simulink model "ForEach6"  (R2017b)
settings: Solver=ode3  StartTime=0.0  StopTime=10.0  FixedStep=0.200000  RelTol=1e-3  EnableMultiTasking=on
settings Model: Creator=hbourbou  LastModifiedBy=hbourbou
settings DataIOCC: LimitDataPoints=on  SaveFormat=Structure
settings OptimizationCC: LifeSpan=inf
settings DebuggingCC: SFUnexpectedBacktrackingDiag=warning  SFNoUnconditionalDefaultTransitionDiag=warning  SFExecutionAtInitializationDiag=none
settings HardwareCC: ProdBitPerPointer=32  ProdBitPerSizeT=32  ProdBitPerPtrDiffT=32  ProdLargestAtomicFloat=None  ProdIntDivRoundTo=Undefined  ProdEndianess=Unspecified  ProdWordSize=32  ProdHWDeviceType=32-bit Generic
settings ModelReferenceCC: PropagateSignalLabelsOutOfModel=off
settings CodeAppCC: StateflowObjectComments=on
settings GRTTargetCC: TargetLangStandard=C89/C90 (ANSI)  GeneratePreprocessorConditionals=Disable all
settings ConfigComp: CovMetricSettings=dw  CovHtmlReporting=on  CovSaveCumulativeToWorkspaceVar=on  CovSaveSingleToWorkspaceVar=on  CovExternalEMLEnable=off

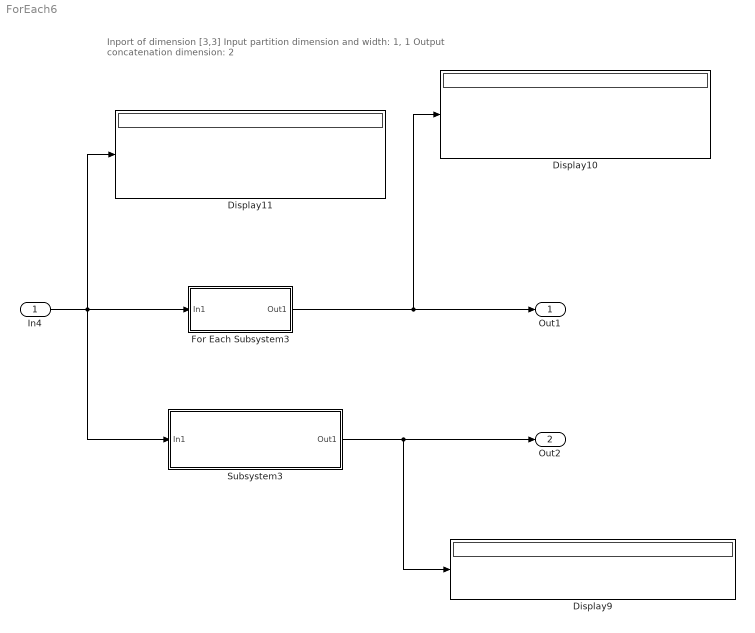
== system ForEach6 ==
  note: Inport of dimension [3,3]
      | Input partition dimension and width: 1, 1
      | Output concatenation dimension: 2
  In4 : Inport  PortDimensions=[3 3]
  Display10 : Display
  Display11 : Display
  Display9 : Display
  For Each Subsystem3 : Subsystem
  Subsystem3 : Subsystem
  Out1 : Outport
  Out2 : Outport  Port=2
  wires:
  In4/1 -> For Each Subsystem3/1(In1), Subsystem3/1(In1), Display11/1
  For Each Subsystem3/1(Out1) -> Out1/1, Display10/1
  Subsystem3/1(Out1) -> Out2/1, Display9/1

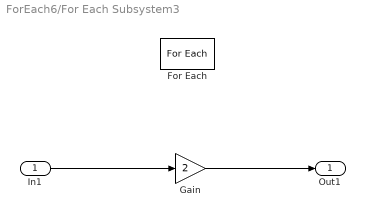
== system ForEach6/For Each Subsystem3 ==
  In1 : Inport  Partition=on  PartitionDimension=1  PartitionWidth=1  PartitionOffset=0
  For Each : ForEach  DisableCoverage=on  IndexMode=One-based
  Gain : Gain  Gain=2
  Out1 : Outport  ConcatenationDimension=2
  wires:
  Gain/1 -> Out1/1
  In1/1 -> Gain/1

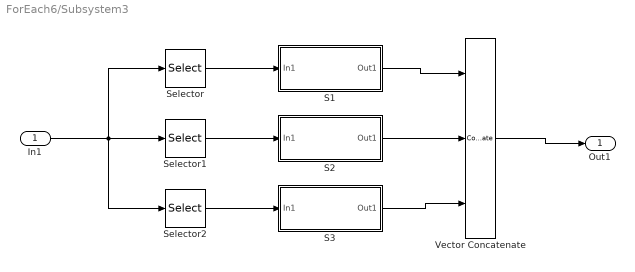
== system ForEach6/Subsystem3 ==
  In1 : Inport
  S1 : Subsystem
  S2 : Subsystem
  S3 : Subsystem
  Selector : Selector  NumberOfDimensions=2  InputPortWidth=3  IndexOptions=Index vector (dialog),Select all  Indices=1,1  OutputSizes=1,1
  Selector1 : Selector  NumberOfDimensions=2  InputPortWidth=3  IndexOptions=Index vector (dialog),Select all  Indices=2,1  OutputSizes=1,1
  Selector2 : Selector  NumberOfDimensions=2  InputPortWidth=3  IndexOptions=Index vector (dialog),Select all  Indices=3,1  OutputSizes=1,1
  Vector Concatenate : Concatenate  NumInputs=3  Mode=Multidimensional array  ConcatenateDimension=2
  Out1 : Outport
  wires:
  S1/1(Out1) -> Vector Concatenate/1
  S3/1(Out1) -> Vector Concatenate/3
  S2/1(Out1) -> Vector Concatenate/2
  Selector/1 -> S1/1(In1)
  Vector Concatenate/1 -> Out1/1
  Selector2/1 -> S3/1(In1)
  Selector1/1 -> S2/1(In1)
  In1/1 -> Selector2/1, Selector1/1, Selector/1

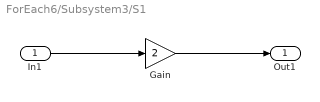
== system ForEach6/Subsystem3/S1 ==
  In1 : Inport
  Gain : Gain  Gain=2
  Out1 : Outport
  wires:
  In1/1 -> Gain/1
  Gain/1 -> Out1/1

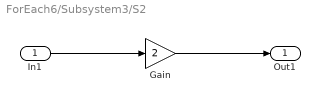
== system ForEach6/Subsystem3/S2 ==
  In1 : Inport
  Gain : Gain  Gain=2
  Out1 : Outport
  wires:
  In1/1 -> Gain/1
  Gain/1 -> Out1/1

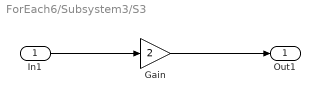
== system ForEach6/Subsystem3/S3 ==
  In1 : Inport
  Gain : Gain  Gain=2
  Out1 : Outport
  wires:
  In1/1 -> Gain/1
  Gain/1 -> Out1/1
